simulink subsystem "Throttle_Controller"  (R2020b)
settings: Solver=VariableStepAuto  StartTime=0.0  StopTime=10.0  RelTol=1e-3
settings Model: Creator=philt  LastModifiedBy=philt

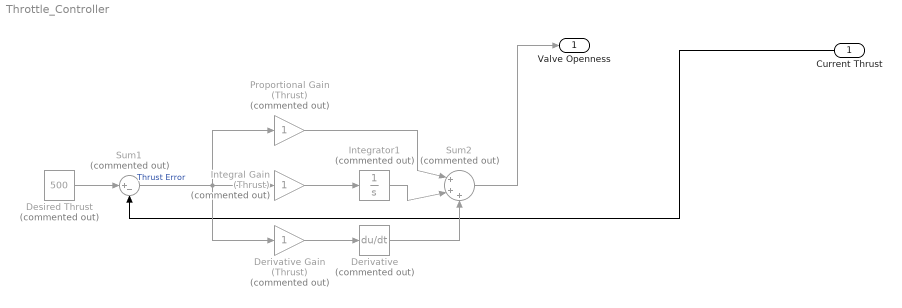
== system Throttle_Controller ==
  Current Thrust : Inport
  Derivative : Derivative  Commented=on
  Derivative Gain (Thrust) : Gain  Commented=on
  Desired Thrust : Constant  Commented=on  Value=500
  Integral Gain (Thrust) : Gain  Commented=on
  Integrator1 : Integrator  Commented=on
  Proportional Gain (Thrust) : Gain  Commented=on
  Sum1 : Sum  Commented=on  Inputs=|+-
  Sum2 : Sum  Commented=on  Inputs=|+++
  Valve Openness : Outport
  wires:
  Sum2/1 -> Valve Openness/1
  Current Thrust/1 -> Sum1/2
  Integral Gain (Thrust)/1 -> Integrator1/1
  Proportional Gain (Thrust)/1 -> Sum2/1
  Integrator1/1 -> Sum2/2
  Derivative Gain (Thrust)/1 -> Derivative/1
  Sum1/1 -> Proportional Gain (Thrust)/1, Derivative Gain (Thrust)/1, Integral Gain (Thrust)/1  "Thrust Error"
  Desired Thrust/1 -> Sum1/1
  Derivative/1 -> Sum2/3
